simulink model "simfivelevelmulti"  (R2023a)
settings: Solver=VariableStepAuto  StartTime=0.0  StopTime=10.0  RelTol=1e-3
libraries: spsIGBTDiodeLib x8, simulink x4, spsDCVoltageSourceLib x2, spsSeriesRLCBranchLib x1, spsVoltageMeasurementLib x1, spspowerguiLib x1
settings Model: Creator=banof  LastModifiedBy=banof

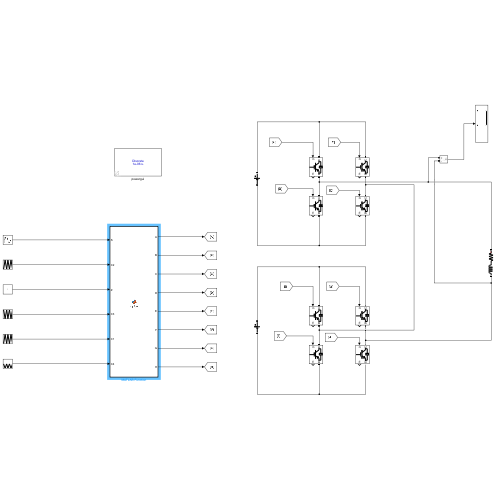
[thumbnail: Simulink's stored preview of the top-level diagram]
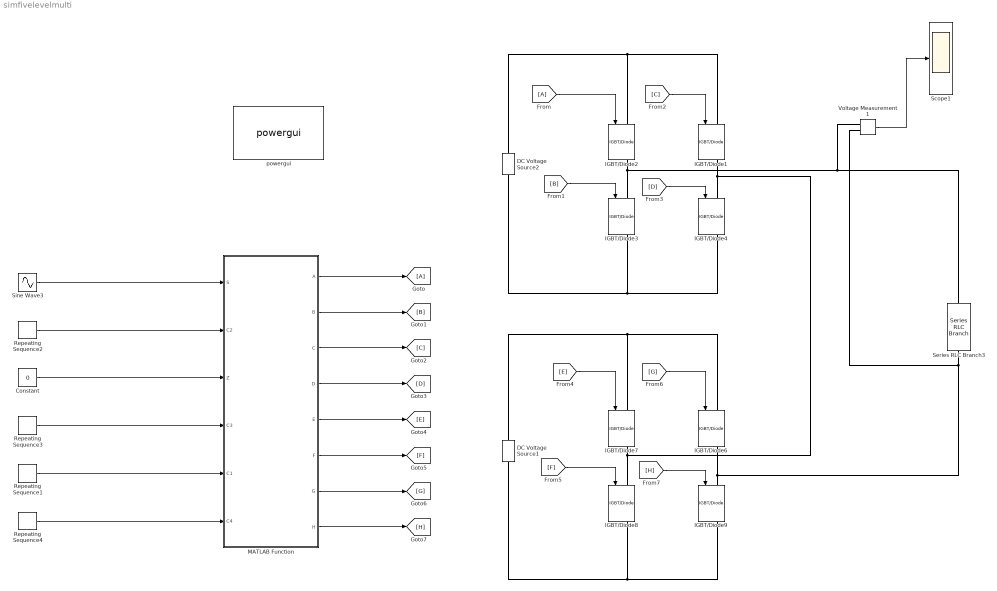
== system simfivelevelmulti ==
  Constant : Constant  Value=0
  DC Voltage Source1 : spsDCVoltageSourceLib/DC Voltage Source  Amplitude=100  Measurements=None
  DC Voltage Source2 : spsDCVoltageSourceLib/DC Voltage Source  Amplitude=100  Measurements=None
  From : From
  Goto : Goto
  IGBT/Diode{1..4,6..9} (8 alike) : spsIGBTDiodeLib/IGBT//Diode  Ron=1e-3  Rs=1e5  Cs=inf  Measurements=on
  MATLAB Function : MATLAB Function  TreatAsAtomicUnit=on
  Repeating Sequence1 : simulink/Sources/Repeating Sequence  rep_seq_t=[0 0.5/1000 1/1000]  rep_seq_y=[0.5 1 0.5]
  Repeating Sequence2 : simulink/Sources/Repeating Sequence  rep_seq_t=[0 0.5/1000 1/1000]  rep_seq_y=[0 0.5 0]
  Repeating Sequence3 : simulink/Sources/Repeating Sequence  rep_seq_t=[0 0.5/1000 1/1000]  rep_seq_y=[0 -0.5 0]
  Repeating Sequence4 : simulink/Sources/Repeating Sequence  rep_seq_t=[0 0.5/1000 1/1000]  rep_seq_y=[-0.5 -1 -0.5]
  Scope1 : Scope
  Series RLC Branch3 : spsSeriesRLCBranchLib/Series RLC Branch  LConnTagsString=__new0  RConnTagsString=__new0  BranchType=RL  Resistance=100  Inductance=100e-3  SetiL0=off  InitialCurrent=0  Capacitance=1e-6  Setx0=off  InitialVoltage=0  Measurements=None
  Sine Wave3 : Sin  Frequency=2*pi*50
  Voltage Measurement1 : spsVoltageMeasurementLib/Voltage Measurement  PhasorSimulation=off  OutputType=Complex  PSBequivalent=0
  powergui : spspowerguiLib/powergui  Priority=1  SimulationMode=Discrete  SampleTime=1e-6  frequency=60  Iterations=50  frequencyindice=0  Pbase=100e6  ErrMax=1e-4  UnitsV=kV  UnitsW=MW  buscounter=0  FunctionMessages=off  echomessages=off  EnableUseOfTLC=off  CurrentSourceSwitches=off  DisableSnubberDevices=off  DisableRonSwitches=off  DisableVfSwitches=off  DisplayEquations=off  AutomaticDiscreteSolvers=off  SolverType=Tustin/Backward Euler (TBE)  Interpol=off  ExternalGateDelay=off  methode=off  Ts=100  x0status=blocks  SPID=on  SwTol=0  HookPort=off  NonlinearTolerance=1e-4  nMaxIteration=100  ContinueOnMaxIteration=off  RestoreLinks=warning  ResistiveCurrentMeasurement=off  Frange=[0:2:500]  Ylog=off  Xlog=on  ShowGrid=off  save=off  variable=ZData  structure=0  ZoomFFT=off  StartTime=0.0  cycles=1  DisplayStyle=1  fundamental=60  FreqAxis=off  MaxFrequency=1000  frequencyindicesteady=1  RmsSteady=1  display=off
  wires:
  MATLAB Function/2(B) -> [B]
  MATLAB Function/8(H) -> [H]
  MATLAB Function/3(C) -> [C]
  MATLAB Function/1(A) -> Goto/1
  MATLAB Function/5(E) -> [E]
  Constant/1 -> MATLAB Function/3(Z)
  Repeating Sequence4/1 -> MATLAB Function/6(C4)
  Repeating Sequence1/1 -> MATLAB Function/5(C1)
  Repeating Sequence3/1 -> MATLAB Function/4(C3)
  Repeating Sequence2/1 -> MATLAB Function/2(C2)
  MATLAB Function/7(G) -> [G]
  MATLAB Function/4(D) -> [D]
  Sine Wave3/1 -> MATLAB Function/1(S)
  MATLAB Function/6(F) -> [F]
  Voltage Measurement1/1 -> Scope1/1
  From/1 -> IGBT/Diode2/1
  [B] -> IGBT/Diode3/1
  [C] -> IGBT/Diode1/1
  [D] -> IGBT/Diode4/1
  [E] -> IGBT/Diode7/1
  [F] -> IGBT/Diode8/1
  [G] -> IGBT/Diode6/1
  [H] -> IGBT/Diode9/1
  connections:
  IGBT/Diode3/RConn1 -- DC Voltage Source2/LConn1 -- IGBT/Diode4/RConn1
  IGBT/Diode9/LConn1 -- Voltage Measurement1/LConn2 -- Series RLC Branch3/RConn1 -- IGBT/Diode6/RConn1
  IGBT/Diode8/RConn1 -- DC Voltage Source1/LConn1 -- IGBT/Diode9/RConn1
  IGBT/Diode2/RConn1 -- Voltage Measurement1/LConn1 -- Series RLC Branch3/LConn1 -- IGBT/Diode3/LConn1
  DC Voltage Source1/RConn1 -- IGBT/Diode7/LConn1 -- IGBT/Diode6/LConn1
  DC Voltage Source2/RConn1 -- IGBT/Diode2/LConn1 -- IGBT/Diode1/LConn1
  IGBT/Diode7/RConn1 -- IGBT/Diode4/LConn1 -- IGBT/Diode1/RConn1 -- IGBT/Diode8/LConn1

== matlab function simfivelevelmulti/MATLAB Function ==
  data: S input; C2 input; A output; B output; C output; D output; E output; F output; G output; H output; Z input; C3 input; C1 input; C4 input
function [A,B,C,D,E,F,G,H]= myfcn(S,C2,Z,C3,C1,C4)
    a=0;b=0;c=0;d=0;e=0;f=0;g=0;h=0;
    if S>C2&&S>Z&&S>C1%2Vdc
    a=1;
    b=0;
    c=0;
    d=1;
    e=1;
    f=0;
    g=0;
    h=1;
elseif S<C1&&S>Z&&S>C2%Vdc
    a=1;
    b=0;
    c=0;
    d=1;
    e=1;
    f=0;
    g=1;
    h=0;
    elseif S<C1&&S>Z&&S<C2%0VDC
   a=1;
   b=0;
    c=1;
    d=0;
    e=1;
    f=0;
    g=1;
    h=0;  
  elseif S>C3&&S<Z&&S>C4%0Vdc
    a=1;
    b=0;
    c=1;
    d=0;
    e=1;
    f=0;
    g=1;
    h=0;    
elseif S<C3&&S>C4&&S<Z%-Vdc
    a=0;
    b=1;
    c=1;
    d=0; 
    e=0;
    f=1;
    g=0;
    h=1;
elseif S<C3&&S<Z&&S<C4%-2Vdc
    a=0;
    b=1;
    c=1;
    d=0;
    e=0;
    f=1;
    g=1;
    h=0;
    end
A=a;
B=b;
C=c;
D=d;
E=e;
F=f;
G=g;
H=h;
